simulink model "LAB_03_SCALARE"  (R2022b)
settings: Solver=ode4  StartTime=0.0  StopTime=100.0  FixedStep=0.1  RelTol=1e-3
values from neighbouring files (symbols this model uses):
  Ir = diag([0, 0, Ir_value])    [LAB_03_3_OCT_MAT_EUL_DOUBLESPIN.m]
  Iy = 0.055    [LAB_03_3_OCT_MAT_EUL.m]    (also in LAB_03_3_OCT_MAT_EUL_2_VERIFICATION.m; LAB_03_3_OCT_MAT_EUL_DOUBLESPIN.m; LAB_03_3_OCT_MAT_EUL_SPINAXIS.m; LAB_03_3_OCT_MAT_EUL_VECT.m)
  Iz = 0.025    [LAB_03_3_OCT_MAT_EUL.m]    (also in LAB_03_3_OCT_MAT_EUL_2_VERIFICATION.m = 0.07; LAB_03_3_OCT_MAT_EUL_DOUBLESPIN.m; LAB_03_3_OCT_MAT_EUL_SPINAXIS.m = 0.07; LAB_03_3_OCT_MAT_EUL_VECT.m)
  om_x0 = 0.45    [LAB_03_3_OCT_MAT_EUL.m]    (also in LAB_03_3_OCT_MAT_EUL_2_VERIFICATION.m = 6.28318530718; LAB_03_3_OCT_MAT_EUL_DOUBLESPIN.m = 1e-06; LAB_03_3_OCT_MAT_EUL_SPINAXIS.m = 0.1; LAB_03_3_OCT_MAT_EUL_VECT.m)
  om_y0 = 0.52    [LAB_03_3_OCT_MAT_EUL.m]    (also in LAB_03_3_OCT_MAT_EUL_2_VERIFICATION.m = 0; LAB_03_3_OCT_MAT_EUL_DOUBLESPIN.m = 1e-06; LAB_03_3_OCT_MAT_EUL_SPINAXIS.m = 6.28318530718; LAB_03_3_OCT_MAT_EUL_VECT.m)
  om_z0 = 0.55    [LAB_03_3_OCT_MAT_EUL.m]    (also in LAB_03_3_OCT_MAT_EUL_2_VERIFICATION.m = 0; LAB_03_3_OCT_MAT_EUL_DOUBLESPIN.m = 0.02; LAB_03_3_OCT_MAT_EUL_SPINAXIS.m = 0.1; LAB_03_3_OCT_MAT_EUL_VECT.m)
  Tw = [0; 0; 0]    [LAB_03_3_OCT_MAT_EUL_DOUBLESPIN.m]
undefined symbols (not defined in the file or in its folder): om_r
settings Model: Creator=maria  LastModifiedBy=maria

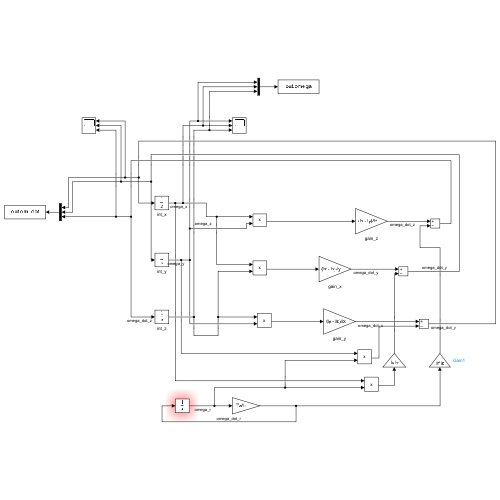
[thumbnail: Simulink's stored preview of the top-level diagram]
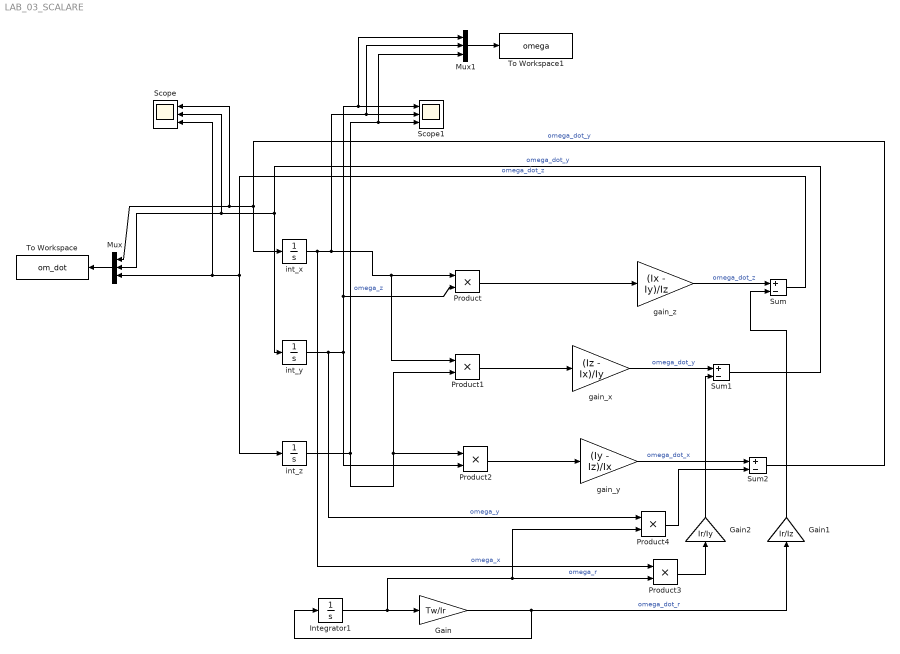
== system LAB_03_SCALARE ==
  Gain : Gain  Gain=Tw/Ir
  Gain1 : Gain  Gain=Ir/Iz
  Gain2 : Gain  Gain=Ir/Iy
  Integrator1 : Integrator  InitialCondition=om_r
  Mux : Mux  Inputs=3
  Mux1 : Mux  Inputs=3
  Product{,1..4} (5 alike) : Product
  Scope : Scope  NumInputPorts=3
  Scope1 : Scope  NumInputPorts=3
  Sum : Sum  Inputs=+-
  Sum1 : Sum  Inputs=+-
  Sum2 : Sum  Inputs=+-
  To Workspace : ToWorkspace  VariableName=om_dot  SampleTime=-1
  To Workspace1 : ToWorkspace  VariableName=omega  SampleTime=-1
  gain_x : Gain  Gain=(Iz - Ix)/Iy
  gain_y : Gain  Gain=(Iy - Iz)/Ix
  gain_z : Gain  Gain=(Ix - Iy)/Iz
  int_x : Integrator  InitialCondition=om_x0
  int_y : Integrator  InitialCondition=om_y0
  int_z : Integrator  InitialCondition=om_z0
  wires:
  Mux/1 -> To Workspace/1
  Product1/1 -> gain_x/1
  Product/1 -> gain_z/1
  Product2/1 -> gain_y/1
  int_x/1 -> Product3/1, Mux1/2, Scope1/2, Product1/1, Product/1  "omega_x"
  int_z/1 -> Mux1/3, Scope1/3, Product1/2, Product2/1  "omega_z"
  int_y/1 -> Product4/1, Mux1/1, Scope1/1, Product/2, Product2/2  "omega_y"
  Sum/1 -> Scope/3, Mux/3, int_z/1  "omega_dot_z"
  Integrator1/1 -> Product4/2, Product3/2, Gain/1  "omega_r"
  Gain/1 -> Gain1/1, Integrator1/1  "omega_dot_r"
  gain_z/1 -> Sum/1  "omega_dot_z"
  Gain1/1 -> Sum/2
  gain_x/1 -> Sum1/1  "omega_dot_y"
  Product3/1 -> Gain2/1
  Gain2/1 -> Sum1/2
  Sum1/1 -> Scope/2, Mux/2, int_y/1  "omega_dot_y"
  Product4/1 -> Sum2/2
  gain_y/1 -> Sum2/1  "omega_dot_x"
  Sum2/1 -> int_x/1, Scope/1, Mux/1  "omega_dot_y"
  Mux1/1 -> To Workspace1/1
